simulink model "Main_C0_C3"  (R2023a)
settings: Solver=ode15s  StartTime=0.0  StopTime=1  RelTol=1e-3
model workspace (MAT data in the model file):
  C_IVD = 0.05
  E_IVD1 = 2.1
  E_IVD2 = 2.2
  E_IVD3 = 1.1
  E_IVD4 = 1.7
  E_IVD5 = 3.2
  IVD1 : object (value not decoded)
  IVD2 : object (value not decoded)
  IVD3 : object (value not decoded)
  IVD4 : object (value not decoded)
  IVD5 : object (value not decoded)
  eo_color = [1 0 0]
  io_color = [0 1 0]
  longissimus_color = [1 0 1]
  multifidus_color = [0 1 1]
  muscle_radius = 1
  psoas_color = [0 0 1]
  ra_color = [1 1 0.5]
symbols that are objects in the model workspace (value not decoded): IVD1, IVD2, IVD3, IVD4, IVD5
undefined symbols (not defined in the file or in its folder): AbdFlex, E_TLFflex, IAP_activation_AbdFlex, IAP_Pa, LeftAbdominalMuscleForce, LeftBackMuscleForce, LeftTransverse1MuscleForce, LeftTransverse2MuscleForce, RightAbdominalMuscleForce, RightBackMuscleForce, RightTransverse1MuscleForce, RightTransverse2MuscleForce, TLFflex2, X, Y, Z
libraries: nesl_utility x1235, sm_lib x960, fl_lib x6, simulink_extras x2
(part 33 of 37)

== matlab function Main_C0_C3/Supraspinous Ligaments/SSL Visualization/Ligament3/MATLAB Function2 ==
  data: x1 input; length output; y1 input; z1 input; x2 input; y2 input; z2 input; Rx output; Ry output; Rz output
function [length, Rx, Ry, Rz] = computeCylinderParameters(x1, y1, z1, x2, y2, z2)
    % Compute the vector between the two frames
    vector = [x2 - x1, y2 - y1, z2 - z1];
    
    % Compute the length of the cylinder
    length = norm(vector);
    
    % Normalize the vector for direction
    unit_vector = vector / length;
    
    % Assume fixed axis (Z-axis)
    fixed_axis = [0, 0, 1];
    
    % Compute the axis of rotation (cross product)
    axis_of_rotation = cross(unit_vector, fixed_axis);
    
    % Avoid division by zero in case vectors are parallel
    if norm(axis_of_rotation) == 0
        % Handle case when the vectors are parallel
        if dot(unit_vector, fixed_axis) > 0
            % Vectors are aligned, no rotation needed
            Rx = 0;
            Ry = 0;
            Rz = 0;
        else
            % Vectors are in opposite directions, 180 degree rotation
            Rx = pi;
            Ry = 0;
            Rz = 0;
        end
        return;
    end
    
    % Normalize the axis of rotation
    axis_of_rotation = axis_of_rotation / norm(axis_of_rotation);
    
    % Compute the angle between vectors (dot product)
    cos_theta = dot(unit_vector, fixed_axis);
    
    % Clamp cos_theta to the range [-1, 1] to avoid domain errors in acos
    cos_theta = max(min(cos_theta, 1), -1);
    angle = acos(cos_theta);  % The angle between the vectors
    
    % Rodrigues' rotation formula to compute the rotation matrix
    K = [0, -axis_of_rotation(3), axis_of_rotation(2); 
         axis_of_rotation(3), 0, -axis_of_rotation(1); 
         -axis_of_rotation(2), axis_of_rotation(1), 0]; 
    R = eye(3) + sin(angle)*K + (1 - cos(angle))*(K^2);
    
    % Now, decompose the rotation matrix to extract the Euler angles
    Rx = -atan2(R(3,2), R(3,3)); % Rotation about X-axis
    %Ry = atan2(-R(3,1), sqrt(R(3,2)^2 + R(3,3)^2)); % Rotation about Y-axis
    denominator = max(sqrt(R(3,2)^2 + R(3,3)^2), eps); % Avoid division by zero
    Ry = -atan2(-R(3,1), denominator);

    
    
    Rz = 0; % No additional rotation needed around the Z-axis
end

== matlab function Main_C0_C3/Muscle Forces/Muscle Visualization/Psoas Visualization/Muscle8/MATLAB Function2 ==
  data: x1 input; length output; y1 input; z1 input; x2 input; y2 input; z2 input; Rx output; Ry output; Rz output
function [length, Rx, Ry, Rz] = computeCylinderParameters(x1, y1, z1, x2, y2, z2)
    % Compute the vector between the two frames
    vector = [x2 - x1, y2 - y1, z2 - z1];
    
    % Compute the length of the cylinder
    length = norm(vector);
    
    % Normalize the vector for direction
    unit_vector = vector / length;
    
    % Assume fixed axis (Z-axis)
    fixed_axis = [0, 0, 1];
    
    % Compute the axis of rotation (cross product)
    axis_of_rotation = cross(unit_vector, fixed_axis);
    
    % Avoid division by zero in case vectors are parallel
    if norm(axis_of_rotation) == 0
        % Handle case when the vectors are parallel
        if dot(unit_vector, fixed_axis) > 0
            % Vectors are aligned, no rotation needed
            Rx = 0;
            Ry = 0;
            Rz = 0;
        else
            % Vectors are in opposite directions, 180 degree rotation
            Rx = pi;
            Ry = 0;
            Rz = 0;
        end
        return;
    end
    
    % Normalize the axis of rotation
    axis_of_rotation = axis_of_rotation / norm(axis_of_rotation);
    
    % Compute the angle between vectors (dot product)
    cos_theta = dot(unit_vector, fixed_axis);
    
    % Clamp cos_theta to the range [-1, 1] to avoid domain errors in acos
    cos_theta = max(min(cos_theta, 1), -1);
    angle = acos(cos_theta);  % The angle between the vectors
    
    % Rodrigues' rotation formula to compute the rotation matrix
    K = [0, -axis_of_rotation(3), axis_of_rotation(2); 
         axis_of_rotation(3), 0, -axis_of_rotation(1); 
         -axis_of_rotation(2), axis_of_rotation(1), 0]; 
    R = eye(3) + sin(angle)*K + (1 - cos(angle))*(K^2);
    
    % Now, decompose the rotation matrix to extract the Euler angles
    Rx = -atan2(R(3,2), R(3,3)); % Rotation about X-axis
    %Ry = atan2(-R(3,1), sqrt(R(3,2)^2 + R(3,3)^2)); % Rotation about Y-axis
    denominator = max(sqrt(R(3,2)^2 + R(3,3)^2), eps); % Avoid division by zero
    Ry = -atan2(-R(3,1), denominator);

    
    
    Rz = 0; % No additional rotation needed around the Z-axis
end

== matlab function Main_C0_C3/Supraspinous Ligaments/SSL Visualization/Ligament4/MATLAB Function2 ==
  data: x1 input; length output; y1 input; z1 input; x2 input; y2 input; z2 input; Rx output; Ry output; Rz output
function [length, Rx, Ry, Rz] = computeCylinderParameters(x1, y1, z1, x2, y2, z2)
    % Compute the vector between the two frames
    vector = [x2 - x1, y2 - y1, z2 - z1];
    
    % Compute the length of the cylinder
    length = norm(vector);
    
    % Normalize the vector for direction
    unit_vector = vector / length;
    
    % Assume fixed axis (Z-axis)
    fixed_axis = [0, 0, 1];
    
    % Compute the axis of rotation (cross product)
    axis_of_rotation = cross(unit_vector, fixed_axis);
    
    % Avoid division by zero in case vectors are parallel
    if norm(axis_of_rotation) == 0
        % Handle case when the vectors are parallel
        if dot(unit_vector, fixed_axis) > 0
            % Vectors are aligned, no rotation needed
            Rx = 0;
            Ry = 0;
            Rz = 0;
        else
            % Vectors are in opposite directions, 180 degree rotation
            Rx = pi;
            Ry = 0;
            Rz = 0;
        end
        return;
    end
    
    % Normalize the axis of rotation
    axis_of_rotation = axis_of_rotation / norm(axis_of_rotation);
    
    % Compute the angle between vectors (dot product)
    cos_theta = dot(unit_vector, fixed_axis);
    
    % Clamp cos_theta to the range [-1, 1] to avoid domain errors in acos
    cos_theta = max(min(cos_theta, 1), -1);
    angle = acos(cos_theta);  % The angle between the vectors
    
    % Rodrigues' rotation formula to compute the rotation matrix
    K = [0, -axis_of_rotation(3), axis_of_rotation(2); 
         axis_of_rotation(3), 0, -axis_of_rotation(1); 
         -axis_of_rotation(2), axis_of_rotation(1), 0]; 
    R = eye(3) + sin(angle)*K + (1 - cos(angle))*(K^2);
    
    % Now, decompose the rotation matrix to extract the Euler angles
    Rx = -atan2(R(3,2), R(3,3)); % Rotation about X-axis
    %Ry = atan2(-R(3,1), sqrt(R(3,2)^2 + R(3,3)^2)); % Rotation about Y-axis
    denominator = max(sqrt(R(3,2)^2 + R(3,3)^2), eps); % Avoid division by zero
    Ry = -atan2(-R(3,1), denominator);

    
    
    Rz = 0; % No additional rotation needed around the Z-axis
end

== matlab function Main_C0_C3/Left and Right Intertransverse Ligaments/ITL Visualization - debug/Ligament3/MATLAB Function2 ==
  data: x1 input; length output; y1 input; z1 input; x2 input; y2 input; z2 input; Rx output; Ry output; Rz output
function [length, Rx, Ry, Rz] = computeCylinderParameters(x1, y1, z1, x2, y2, z2)
    % Compute the vector between the two frames
    vector = [x2 - x1, y2 - y1, z2 - z1];
    
    % Compute the length of the cylinder
    length = norm(vector);
    
    % Normalize the vector for direction
    unit_vector = vector / length;
    
    % Assume fixed axis (Z-axis)
    fixed_axis = [0, 0, 1];
    
    % Compute the axis of rotation (cross product)
    axis_of_rotation = cross(unit_vector, fixed_axis);
    
    % Avoid division by zero in case vectors are parallel
    if norm(axis_of_rotation) == 0
        % Handle case when the vectors are parallel
        if dot(unit_vector, fixed_axis) > 0
            % Vectors are aligned, no rotation needed
            Rx = 0;
            Ry = 0;
            Rz = 0;
        else
            % Vectors are in opposite directions, 180 degree rotation
            Rx = pi;
            Ry = 0;
            Rz = 0;
        end
        return;
    end
    
    % Normalize the axis of rotation
    axis_of_rotation = axis_of_rotation / norm(axis_of_rotation);
    
    % Compute the angle between vectors (dot product)
    cos_theta = dot(unit_vector, fixed_axis);
    
    % Clamp cos_theta to the range [-1, 1] to avoid domain errors in acos
    cos_theta = max(min(cos_theta, 1), -1);
    angle = acos(cos_theta);  % The angle between the vectors
    
    % Rodrigues' rotation formula to compute the rotation matrix
    K = [0, -axis_of_rotation(3), axis_of_rotation(2); 
         axis_of_rotation(3), 0, -axis_of_rotation(1); 
         -axis_of_rotation(2), axis_of_rotation(1), 0]; 
    R = eye(3) + sin(angle)*K + (1 - cos(angle))*(K^2);
    
    % Now, decompose the rotation matrix to extract the Euler angles
    Rx = -atan2(R(3,2), R(3,3)); % Rotation about X-axis
    %Ry = atan2(-R(3,1), sqrt(R(3,2)^2 + R(3,3)^2)); % Rotation about Y-axis
    denominator = max(sqrt(R(3,2)^2 + R(3,3)^2), eps); % Avoid division by zero
    Ry = -atan2(-R(3,1), denominator);

    
    
    Rz = 0; % No additional rotation needed around the Z-axis
end

== matlab function Main_C0_C3/Left and Right Intertransverse Ligaments/ITL Visualization - debug/Ligament1/MATLAB Function2 ==
  data: x1 input; length output; y1 input; z1 input; x2 input; y2 input; z2 input; Rx output; Ry output; Rz output
function [length, Rx, Ry, Rz] = computeCylinderParameters(x1, y1, z1, x2, y2, z2)
    % Compute the vector between the two frames
    vector = [x2 - x1, y2 - y1, z2 - z1];
    
    % Compute the length of the cylinder
    length = norm(vector);
    
    % Normalize the vector for direction
    unit_vector = vector / length;
    
    % Assume fixed axis (Z-axis)
    fixed_axis = [0, 0, 1];
    
    % Compute the axis of rotation (cross product)
    axis_of_rotation = cross(unit_vector, fixed_axis);
    
    % Avoid division by zero in case vectors are parallel
    if norm(axis_of_rotation) == 0
        % Handle case when the vectors are parallel
        if dot(unit_vector, fixed_axis) > 0
            % Vectors are aligned, no rotation needed
            Rx = 0;
            Ry = 0;
            Rz = 0;
        else
            % Vectors are in opposite directions, 180 degree rotation
            Rx = pi;
            Ry = 0;
            Rz = 0;
        end
        return;
    end
    
    % Normalize the axis of rotation
    axis_of_rotation = axis_of_rotation / norm(axis_of_rotation);
    
    % Compute the angle between vectors (dot product)
    cos_theta = dot(unit_vector, fixed_axis);
    
    % Clamp cos_theta to the range [-1, 1] to avoid domain errors in acos
    cos_theta = max(min(cos_theta, 1), -1);
    angle = acos(cos_theta);  % The angle between the vectors
    
    % Rodrigues' rotation formula to compute the rotation matrix
    K = [0, -axis_of_rotation(3), axis_of_rotation(2); 
         axis_of_rotation(3), 0, -axis_of_rotation(1); 
         -axis_of_rotation(2), axis_of_rotation(1), 0]; 
    R = eye(3) + sin(angle)*K + (1 - cos(angle))*(K^2);
    
    % Now, decompose the rotation matrix to extract the Euler angles
    Rx = -atan2(R(3,2), R(3,3)); % Rotation about X-axis
    %Ry = atan2(-R(3,1), sqrt(R(3,2)^2 + R(3,3)^2)); % Rotation about Y-axis
    denominator = max(sqrt(R(3,2)^2 + R(3,3)^2), eps); % Avoid division by zero
    Ry = -atan2(-R(3,1), denominator);

    
    
    Rz = 0; % No additional rotation needed around the Z-axis
end

== matlab function Main_C0_C3/Left and Right Intertransverse Ligaments/ITL Visualization - debug/Ligament2/MATLAB Function2 ==
  data: x1 input; length output; y1 input; z1 input; x2 input; y2 input; z2 input; Rx output; Ry output; Rz output
function [length, Rx, Ry, Rz] = computeCylinderParameters(x1, y1, z1, x2, y2, z2)
    % Compute the vector between the two frames
    vector = [x2 - x1, y2 - y1, z2 - z1];
    
    % Compute the length of the cylinder
    length = norm(vector);
    
    % Normalize the vector for direction
    unit_vector = vector / length;
    
    % Assume fixed axis (Z-axis)
    fixed_axis = [0, 0, 1];
    
    % Compute the axis of rotation (cross product)
    axis_of_rotation = cross(unit_vector, fixed_axis);
    
    % Avoid division by zero in case vectors are parallel
    if norm(axis_of_rotation) == 0
        % Handle case when the vectors are parallel
        if dot(unit_vector, fixed_axis) > 0
            % Vectors are aligned, no rotation needed
            Rx = 0;
            Ry = 0;
            Rz = 0;
        else
            % Vectors are in opposite directions, 180 degree rotation
            Rx = pi;
            Ry = 0;
            Rz = 0;
        end
        return;
    end
    
    % Normalize the axis of rotation
    axis_of_rotation = axis_of_rotation / norm(axis_of_rotation);
    
    % Compute the angle between vectors (dot product)
    cos_theta = dot(unit_vector, fixed_axis);
    
    % Clamp cos_theta to the range [-1, 1] to avoid domain errors in acos
    cos_theta = max(min(cos_theta, 1), -1);
    angle = acos(cos_theta);  % The angle between the vectors
    
    % Rodrigues' rotation formula to compute the rotation matrix
    K = [0, -axis_of_rotation(3), axis_of_rotation(2); 
         axis_of_rotation(3), 0, -axis_of_rotation(1); 
         -axis_of_rotation(2), axis_of_rotation(1), 0]; 
    R = eye(3) + sin(angle)*K + (1 - cos(angle))*(K^2);
    
    % Now, decompose the rotation matrix to extract the Euler angles
    Rx = -atan2(R(3,2), R(3,3)); % Rotation about X-axis
    %Ry = atan2(-R(3,1), sqrt(R(3,2)^2 + R(3,3)^2)); % Rotation about Y-axis
    denominator = max(sqrt(R(3,2)^2 + R(3,3)^2), eps); % Avoid division by zero
    Ry = -atan2(-R(3,1), denominator);

    
    
    Rz = 0; % No additional rotation needed around the Z-axis
end

== matlab function Main_C0_C3/Left and Right Intertransverse Ligaments/ITL Visualization - debug/Ligament4/MATLAB Function2 ==
  data: x1 input; length output; y1 input; z1 input; x2 input; y2 input; z2 input; Rx output; Ry output; Rz output
function [length, Rx, Ry, Rz] = computeCylinderParameters(x1, y1, z1, x2, y2, z2)
    % Compute the vector between the two frames
    vector = [x2 - x1, y2 - y1, z2 - z1];
    
    % Compute the length of the cylinder
    length = norm(vector);
    
    % Normalize the vector for direction
    unit_vector = vector / length;
    
    % Assume fixed axis (Z-axis)
    fixed_axis = [0, 0, 1];
    
    % Compute the axis of rotation (cross product)
    axis_of_rotation = cross(unit_vector, fixed_axis);
    
    % Avoid division by zero in case vectors are parallel
    if norm(axis_of_rotation) == 0
        % Handle case when the vectors are parallel
        if dot(unit_vector, fixed_axis) > 0
            % Vectors are aligned, no rotation needed
            Rx = 0;
            Ry = 0;
            Rz = 0;
        else
            % Vectors are in opposite directions, 180 degree rotation
            Rx = pi;
            Ry = 0;
            Rz = 0;
        end
        return;
    end
    
    % Normalize the axis of rotation
    axis_of_rotation = axis_of_rotation / norm(axis_of_rotation);
    
    % Compute the angle between vectors (dot product)
    cos_theta = dot(unit_vector, fixed_axis);
    
    % Clamp cos_theta to the range [-1, 1] to avoid domain errors in acos
    cos_theta = max(min(cos_theta, 1), -1);
    angle = acos(cos_theta);  % The angle between the vectors
    
    % Rodrigues' rotation formula to compute the rotation matrix
    K = [0, -axis_of_rotation(3), axis_of_rotation(2); 
         axis_of_rotation(3), 0, -axis_of_rotation(1); 
         -axis_of_rotation(2), axis_of_rotation(1), 0]; 
    R = eye(3) + sin(angle)*K + (1 - cos(angle))*(K^2);
    
    % Now, decompose the rotation matrix to extract the Euler angles
    Rx = -atan2(R(3,2), R(3,3)); % Rotation about X-axis
    %Ry = atan2(-R(3,1), sqrt(R(3,2)^2 + R(3,3)^2)); % Rotation about Y-axis
    denominator = max(sqrt(R(3,2)^2 + R(3,3)^2), eps); % Avoid division by zero
    Ry = -atan2(-R(3,1), denominator);

    
    
    Rz = 0; % No additional rotation needed around the Z-axis
end

== matlab function Main_C0_C3/Left and Right Intertransverse Ligaments/ITL Visualization - debug/Ligament5/MATLAB Function2 ==
  data: x1 input; length output; y1 input; z1 input; x2 input; y2 input; z2 input; Rx output; Ry output; Rz output
function [length, Rx, Ry, Rz] = computeCylinderParameters(x1, y1, z1, x2, y2, z2)
    % Compute the vector between the two frames
    vector = [x2 - x1, y2 - y1, z2 - z1];
    
    % Compute the length of the cylinder
    length = norm(vector);
    
    % Normalize the vector for direction
    unit_vector = vector / length;
    
    % Assume fixed axis (Z-axis)
    fixed_axis = [0, 0, 1];
    
    % Compute the axis of rotation (cross product)
    axis_of_rotation = cross(unit_vector, fixed_axis);
    
    % Avoid division by zero in case vectors are parallel
    if norm(axis_of_rotation) == 0
        % Handle case when the vectors are parallel
        if dot(unit_vector, fixed_axis) > 0
            % Vectors are aligned, no rotation needed
            Rx = 0;
            Ry = 0;
            Rz = 0;
        else
            % Vectors are in opposite directions, 180 degree rotation
            Rx = pi;
            Ry = 0;
            Rz = 0;
        end
        return;
    end
    
    % Normalize the axis of rotation
    axis_of_rotation = axis_of_rotation / norm(axis_of_rotation);
    
    % Compute the angle between vectors (dot product)
    cos_theta = dot(unit_vector, fixed_axis);
    
    % Clamp cos_theta to the range [-1, 1] to avoid domain errors in acos
    cos_theta = max(min(cos_theta, 1), -1);
    angle = acos(cos_theta);  % The angle between the vectors
    
    % Rodrigues' rotation formula to compute the rotation matrix
    K = [0, -axis_of_rotation(3), axis_of_rotation(2); 
         axis_of_rotation(3), 0, -axis_of_rotation(1); 
         -axis_of_rotation(2), axis_of_rotation(1), 0]; 
    R = eye(3) + sin(angle)*K + (1 - cos(angle))*(K^2);
    
    % Now, decompose the rotation matrix to extract the Euler angles
    Rx = -atan2(R(3,2), R(3,3)); % Rotation about X-axis
    %Ry = atan2(-R(3,1), sqrt(R(3,2)^2 + R(3,3)^2)); % Rotation about Y-axis
    denominator = max(sqrt(R(3,2)^2 + R(3,3)^2), eps); % Avoid division by zero
    Ry = -atan2(-R(3,1), denominator);

    
    
    Rz = 0; % No additional rotation needed around the Z-axis
end

== matlab function Main_C0_C3/Left and Right Intertransverse Ligaments/ITL Visualization - debug/Ligament6/MATLAB Function2 ==
  data: x1 input; length output; y1 input; z1 input; x2 input; y2 input; z2 input; Rx output; Ry output; Rz output
function [length, Rx, Ry, Rz] = computeCylinderParameters(x1, y1, z1, x2, y2, z2)
    % Compute the vector between the two frames
    vector = [x2 - x1, y2 - y1, z2 - z1];
    
    % Compute the length of the cylinder
    length = norm(vector);
    
    % Normalize the vector for direction
    unit_vector = vector / length;
    
    % Assume fixed axis (Z-axis)
    fixed_axis = [0, 0, 1];
    
    % Compute the axis of rotation (cross product)
    axis_of_rotation = cross(unit_vector, fixed_axis);
    
    % Avoid division by zero in case vectors are parallel
    if norm(axis_of_rotation) == 0
        % Handle case when the vectors are parallel
        if dot(unit_vector, fixed_axis) > 0
            % Vectors are aligned, no rotation needed
            Rx = 0;
            Ry = 0;
            Rz = 0;
        else
            % Vectors are in opposite directions, 180 degree rotation
            Rx = pi;
            Ry = 0;
            Rz = 0;
        end
        return;
    end
    
    % Normalize the axis of rotation
    axis_of_rotation = axis_of_rotation / norm(axis_of_rotation);
    
    % Compute the angle between vectors (dot product)
    cos_theta = dot(unit_vector, fixed_axis);
    
    % Clamp cos_theta to the range [-1, 1] to avoid domain errors in acos
    cos_theta = max(min(cos_theta, 1), -1);
    angle = acos(cos_theta);  % The angle between the vectors
    
    % Rodrigues' rotation formula to compute the rotation matrix
    K = [0, -axis_of_rotation(3), axis_of_rotation(2); 
         axis_of_rotation(3), 0, -axis_of_rotation(1); 
         -axis_of_rotation(2), axis_of_rotation(1), 0]; 
    R = eye(3) + sin(angle)*K + (1 - cos(angle))*(K^2);
    
    % Now, decompose the rotation matrix to extract the Euler angles
    Rx = -atan2(R(3,2), R(3,3)); % Rotation about X-axis
    %Ry = atan2(-R(3,1), sqrt(R(3,2)^2 + R(3,3)^2)); % Rotation about Y-axis
    denominator = max(sqrt(R(3,2)^2 + R(3,3)^2), eps); % Avoid division by zero
    Ry = -atan2(-R(3,1), denominator);

    
    
    Rz = 0; % No additional rotation needed around the Z-axis
end

== matlab function Main_C0_C3/Left and Right Intertransverse Ligaments/ITL Visualization - debug/Ligament7/MATLAB Function2 ==
  data: x1 input; length output; y1 input; z1 input; x2 input; y2 input; z2 input; Rx output; Ry output; Rz output
function [length, Rx, Ry, Rz] = computeCylinderParameters(x1, y1, z1, x2, y2, z2)
    % Compute the vector between the two frames
    vector = [x2 - x1, y2 - y1, z2 - z1];
    
    % Compute the length of the cylinder
    length = norm(vector);
    
    % Normalize the vector for direction
    unit_vector = vector / length;
    
    % Assume fixed axis (Z-axis)
    fixed_axis = [0, 0, 1];
    
    % Compute the axis of rotation (cross product)
    axis_of_rotation = cross(unit_vector, fixed_axis);
    
    % Avoid division by zero in case vectors are parallel
    if norm(axis_of_rotation) == 0
        % Handle case when the vectors are parallel
        if dot(unit_vector, fixed_axis) > 0
            % Vectors are aligned, no rotation needed
            Rx = 0;
            Ry = 0;
            Rz = 0;
        else
            % Vectors are in opposite directions, 180 degree rotation
            Rx = pi;
            Ry = 0;
            Rz = 0;
        end
        return;
    end
    
    % Normalize the axis of rotation
    axis_of_rotation = axis_of_rotation / norm(axis_of_rotation);
    
    % Compute the angle between vectors (dot product)
    cos_theta = dot(unit_vector, fixed_axis);
    
    % Clamp cos_theta to the range [-1, 1] to avoid domain errors in acos
    cos_theta = max(min(cos_theta, 1), -1);
    angle = acos(cos_theta);  % The angle between the vectors
    
    % Rodrigues' rotation formula to compute the rotation matrix
    K = [0, -axis_of_rotation(3), axis_of_rotation(2); 
         axis_of_rotation(3), 0, -axis_of_rotation(1); 
         -axis_of_rotation(2), axis_of_rotation(1), 0]; 
    R = eye(3) + sin(angle)*K + (1 - cos(angle))*(K^2);
    
    % Now, decompose the rotation matrix to extract the Euler angles
    Rx = -atan2(R(3,2), R(3,3)); % Rotation about X-axis
    %Ry = atan2(-R(3,1), sqrt(R(3,2)^2 + R(3,3)^2)); % Rotation about Y-axis
    denominator = max(sqrt(R(3,2)^2 + R(3,3)^2), eps); % Avoid division by zero
    Ry = -atan2(-R(3,1), denominator);

    
    
    Rz = 0; % No additional rotation needed around the Z-axis
end

== matlab function Main_C0_C3/Left and Right Intertransverse Ligaments/ITL Visualization - debug/Ligament8/MATLAB Function2 ==
  data: x1 input; length output; y1 input; z1 input; x2 input; y2 input; z2 input; Rx output; Ry output; Rz output
function [length, Rx, Ry, Rz] = computeCylinderParameters(x1, y1, z1, x2, y2, z2)
    % Compute the vector between the two frames
    vector = [x2 - x1, y2 - y1, z2 - z1];
    
    % Compute the length of the cylinder
    length = norm(vector);
    
    % Normalize the vector for direction
    unit_vector = vector / length;
    
    % Assume fixed axis (Z-axis)
    fixed_axis = [0, 0, 1];
    
    % Compute the axis of rotation (cross product)
    axis_of_rotation = cross(unit_vector, fixed_axis);
    
    % Avoid division by zero in case vectors are parallel
    if norm(axis_of_rotation) == 0
        % Handle case when the vectors are parallel
        if dot(unit_vector, fixed_axis) > 0
            % Vectors are aligned, no rotation needed
            Rx = 0;
            Ry = 0;
            Rz = 0;
        else
            % Vectors are in opposite directions, 180 degree rotation
            Rx = pi;
            Ry = 0;
            Rz = 0;
        end
        return;
    end
    
    % Normalize the axis of rotation
    axis_of_rotation = axis_of_rotation / norm(axis_of_rotation);
    
    % Compute the angle between vectors (dot product)
    cos_theta = dot(unit_vector, fixed_axis);
    
    % Clamp cos_theta to the range [-1, 1] to avoid domain errors in acos
    cos_theta = max(min(cos_theta, 1), -1);
    angle = acos(cos_theta);  % The angle between the vectors
    
    % Rodrigues' rotation formula to compute the rotation matrix
    K = [0, -axis_of_rotation(3), axis_of_rotation(2); 
         axis_of_rotation(3), 0, -axis_of_rotation(1); 
         -axis_of_rotation(2), axis_of_rotation(1), 0]; 
    R = eye(3) + sin(angle)*K + (1 - cos(angle))*(K^2);
    
    % Now, decompose the rotation matrix to extract the Euler angles
    Rx = -atan2(R(3,2), R(3,3)); % Rotation about X-axis
    %Ry = atan2(-R(3,1), sqrt(R(3,2)^2 + R(3,3)^2)); % Rotation about Y-axis
    denominator = max(sqrt(R(3,2)^2 + R(3,3)^2), eps); % Avoid division by zero
    Ry = -atan2(-R(3,1), denominator);

    
    
    Rz = 0; % No additional rotation needed around the Z-axis
end

== matlab function Main_C0_C3/Left and Right Intertransverse Ligaments/ITL Visualization - debug/Ligament9/MATLAB Function2 ==
  data: x1 input; length output; y1 input; z1 input; x2 input; y2 input; z2 input; Rx output; Ry output; Rz output
function [length, Rx, Ry, Rz] = computeCylinderParameters(x1, y1, z1, x2, y2, z2)
    % Compute the vector between the two frames
    vector = [x2 - x1, y2 - y1, z2 - z1];
    
    % Compute the length of the cylinder
    length = norm(vector);
    
    % Normalize the vector for direction
    unit_vector = vector / length;
    
    % Assume fixed axis (Z-axis)
    fixed_axis = [0, 0, 1];
    
    % Compute the axis of rotation (cross product)
    axis_of_rotation = cross(unit_vector, fixed_axis);
    
    % Avoid division by zero in case vectors are parallel
    if norm(axis_of_rotation) == 0
        % Handle case when the vectors are parallel
        if dot(unit_vector, fixed_axis) > 0
            % Vectors are aligned, no rotation needed
            Rx = 0;
            Ry = 0;
            Rz = 0;
        else
            % Vectors are in opposite directions, 180 degree rotation
            Rx = pi;
            Ry = 0;
            Rz = 0;
        end
        return;
    end
    
    % Normalize the axis of rotation
    axis_of_rotation = axis_of_rotation / norm(axis_of_rotation);
    
    % Compute the angle between vectors (dot product)
    cos_theta = dot(unit_vector, fixed_axis);
    
    % Clamp cos_theta to the range [-1, 1] to avoid domain errors in acos
    cos_theta = max(min(cos_theta, 1), -1);
    angle = acos(cos_theta);  % The angle between the vectors
    
    % Rodrigues' rotation formula to compute the rotation matrix
    K = [0, -axis_of_rotation(3), axis_of_rotation(2); 
         axis_of_rotation(3), 0, -axis_of_rotation(1); 
         -axis_of_rotation(2), axis_of_rotation(1), 0]; 
    R = eye(3) + sin(angle)*K + (1 - cos(angle))*(K^2);
    
    % Now, decompose the rotation matrix to extract the Euler angles
    Rx = -atan2(R(3,2), R(3,3)); % Rotation about X-axis
    %Ry = atan2(-R(3,1), sqrt(R(3,2)^2 + R(3,3)^2)); % Rotation about Y-axis
    denominator = max(sqrt(R(3,2)^2 + R(3,3)^2), eps); % Avoid division by zero
    Ry = -atan2(-R(3,1), denominator);

    
    
    Rz = 0; % No additional rotation needed around the Z-axis
end

== matlab function Main_C0_C3/Muscle Forces/Muscle Visualization/Multifidus Visualization/Muscle9/MATLAB Function2 ==
  data: x1 input; length output; y1 input; z1 input; x2 input; y2 input; z2 input; Rx output; Ry output; Rz output
function [length, Rx, Ry, Rz] = computeCylinderParameters(x1, y1, z1, x2, y2, z2)
    % Compute the vector between the two frames
    vector = [x2 - x1, y2 - y1, z2 - z1];
    
    % Compute the length of the cylinder
    length = norm(vector);
    
    % Normalize the vector for direction
    unit_vector = vector / length;
    
    % Assume fixed axis (Z-axis)
    fixed_axis = [0, 0, 1];
    
    % Compute the axis of rotation (cross product)
    axis_of_rotation = cross(unit_vector, fixed_axis);
    
    % Avoid division by zero in case vectors are parallel
    if norm(axis_of_rotation) == 0
        % Handle case when the vectors are parallel
        if dot(unit_vector, fixed_axis) > 0
            % Vectors are aligned, no rotation needed
            Rx = 0;
            Ry = 0;
            Rz = 0;
        else
            % Vectors are in opposite directions, 180 degree rotation
            Rx = pi;
            Ry = 0;
            Rz = 0;
        end
        return;
    end
    
    % Normalize the axis of rotation
    axis_of_rotation = axis_of_rotation / norm(axis_of_rotation);
    
    % Compute the angle between vectors (dot product)
    cos_theta = dot(unit_vector, fixed_axis);
    
    % Clamp cos_theta to the range [-1, 1] to avoid domain errors in acos
    cos_theta = max(min(cos_theta, 1), -1);
    angle = acos(cos_theta);  % The angle between the vectors
    
    % Rodrigues' rotation formula to compute the rotation matrix
    K = [0, -axis_of_rotation(3), axis_of_rotation(2); 
         axis_of_rotation(3), 0, -axis_of_rotation(1); 
         -axis_of_rotation(2), axis_of_rotation(1), 0]; 
    R = eye(3) + sin(angle)*K + (1 - cos(angle))*(K^2);
    
    % Now, decompose the rotation matrix to extract the Euler angles
    Rx = -atan2(R(3,2), R(3,3)); % Rotation about X-axis
    %Ry = atan2(-R(3,1), sqrt(R(3,2)^2 + R(3,3)^2)); % Rotation about Y-axis
    denominator = max(sqrt(R(3,2)^2 + R(3,3)^2), eps); % Avoid division by zero
    Ry = -atan2(-R(3,1), denominator);

    
    
    Rz = 0; % No additional rotation needed around the Z-axis
end

== matlab function Main_C0_C3/Left and Right Intertransverse Ligaments/ITL Visualization - debug/Ligament10/MATLAB Function2 ==
  data: x1 input; length output; y1 input; z1 input; x2 input; y2 input; z2 input; Rx output; Ry output; Rz output
function [length, Rx, Ry, Rz] = computeCylinderParameters(x1, y1, z1, x2, y2, z2)
    % Compute the vector between the two frames
    vector = [x2 - x1, y2 - y1, z2 - z1];
    
    % Compute the length of the cylinder
    length = norm(vector);
    
    % Normalize the vector for direction
    unit_vector = vector / length;
    
    % Assume fixed axis (Z-axis)
    fixed_axis = [0, 0, 1];
    
    % Compute the axis of rotation (cross product)
    axis_of_rotation = cross(unit_vector, fixed_axis);
    
    % Avoid division by zero in case vectors are parallel
    if norm(axis_of_rotation) == 0
        % Handle case when the vectors are parallel
        if dot(unit_vector, fixed_axis) > 0
            % Vectors are aligned, no rotation needed
            Rx = 0;
            Ry = 0;
            Rz = 0;
        else
            % Vectors are in opposite directions, 180 degree rotation
            Rx = pi;
            Ry = 0;
            Rz = 0;
        end
        return;
    end
    
    % Normalize the axis of rotation
    axis_of_rotation = axis_of_rotation / norm(axis_of_rotation);
    
    % Compute the angle between vectors (dot product)
    cos_theta = dot(unit_vector, fixed_axis);
    
    % Clamp cos_theta to the range [-1, 1] to avoid domain errors in acos
    cos_theta = max(min(cos_theta, 1), -1);
    angle = acos(cos_theta);  % The angle between the vectors
    
    % Rodrigues' rotation formula to compute the rotation matrix
    K = [0, -axis_of_rotation(3), axis_of_rotation(2); 
         axis_of_rotation(3), 0, -axis_of_rotation(1); 
         -axis_of_rotation(2), axis_of_rotation(1), 0]; 
    R = eye(3) + sin(angle)*K + (1 - cos(angle))*(K^2);
    
    % Now, decompose the rotation matrix to extract the Euler angles
    Rx = -atan2(R(3,2), R(3,3)); % Rotation about X-axis
    %Ry = atan2(-R(3,1), sqrt(R(3,2)^2 + R(3,3)^2)); % Rotation about Y-axis
    denominator = max(sqrt(R(3,2)^2 + R(3,3)^2), eps); % Avoid division by zero
    Ry = -atan2(-R(3,1), denominator);

    
    
    Rz = 0; % No additional rotation needed around the Z-axis
end

== matlab function Main_C0_C3/TLF Flex/Latissimus Dorsi/WrappedMuscle2/MATLAB Function1 ==
  data: x1 input; length output; y1 input; z1 input; x2 input; y2 input; z2 input; Rx output; Ry output; Rz output
function [length, Rx, Ry, Rz] = computeCylinderParameters(x1, y1, z1, x2, y2, z2)
    % Compute the vector between the two frames
    vector = [x2 - x1, y2 - y1, z2 - z1];
    
    % Compute the length of the cylinder
    length = norm(vector);
    
    % Normalize the vector for direction
    unit_vector = vector / length;
    
    % Assume fixed axis (Z-axis)
    fixed_axis = [0, 0, 1];
    
    % Compute the axis of rotation (cross product)
    axis_of_rotation = cross(unit_vector, fixed_axis);
    
    % Avoid division by zero in case vectors are parallel
    if norm(axis_of_rotation) == 0
        % Handle case when the vectors are parallel
        if dot(unit_vector, fixed_axis) > 0
            % Vectors are aligned, no rotation needed
            Rx = 0;
            Ry = 0;
            Rz = 0;
        else
            % Vectors are in opposite directions, 180 degree rotation
            Rx = pi;
            Ry = 0;
            Rz = 0;
        end
        return;
    end
    
    % Normalize the axis of rotation
    axis_of_rotation = axis_of_rotation / norm(axis_of_rotation);
    
    % Compute the angle between vectors (dot product)
    cos_theta = dot(unit_vector, fixed_axis);
    
    % Clamp cos_theta to the range [-1, 1] to avoid domain errors in acos
    cos_theta = max(min(cos_theta, 1), -1);
    angle = acos(cos_theta);  % The angle between the vectors
    
    % Rodrigues' rotation formula to compute the rotation matrix
    K = [0, -axis_of_rotation(3), axis_of_rotation(2); 
         axis_of_rotation(3), 0, -axis_of_rotation(1); 
         -axis_of_rotation(2), axis_of_rotation(1), 0]; 
    R = eye(3) + sin(angle)*K + (1 - cos(angle))*(K^2);
    
    % Now, decompose the rotation matrix to extract the Euler angles
    Rx = -atan2(R(3,2), R(3,3)); % Rotation about X-axis
    %Ry = atan2(-R(3,1), sqrt(R(3,2)^2 + R(3,3)^2)); % Rotation about Y-axis
    denominator = max(sqrt(R(3,2)^2 + R(3,3)^2), eps); % Avoid division by zero
    Ry = -atan2(-R(3,1), denominator);

    
    
    Rz = 0; % No additional rotation needed around the Z-axis
end

== matlab function Main_C0_C3/TLF Flex/Latissimus Dorsi/WrappedMuscle1/MATLAB Function3 ==
  data: x1 input; length output; y1 input; z1 input; x2 input; y2 input; z2 input; Rx output; Ry output; Rz output
function [length, Rx, Ry, Rz] = computeCylinderParameters(x1, y1, z1, x2, y2, z2)
    % Compute the vector between the two frames
    vector = [x2 - x1, y2 - y1, z2 - z1];
    
    % Compute the length of the cylinder
    length = norm(vector);
    
    % Normalize the vector for direction
    unit_vector = vector / length;
    
    % Assume fixed axis (Z-axis)
    fixed_axis = [0, 0, 1];
    
    % Compute the axis of rotation (cross product)
    axis_of_rotation = cross(unit_vector, fixed_axis);
    
    % Avoid division by zero in case vectors are parallel
    if norm(axis_of_rotation) == 0
        % Handle case when the vectors are parallel
        if dot(unit_vector, fixed_axis) > 0
            % Vectors are aligned, no rotation needed
            Rx = 0;
            Ry = 0;
            Rz = 0;
        else
            % Vectors are in opposite directions, 180 degree rotation
            Rx = pi;
            Ry = 0;
            Rz = 0;
        end
        return;
    end
    
    % Normalize the axis of rotation
    axis_of_rotation = axis_of_rotation / norm(axis_of_rotation);
    
    % Compute the angle between vectors (dot product)
    cos_theta = dot(unit_vector, fixed_axis);
    
    % Clamp cos_theta to the range [-1, 1] to avoid domain errors in acos
    cos_theta = max(min(cos_theta, 1), -1);
    angle = acos(cos_theta);  % The angle between the vectors
    
    % Rodrigues' rotation formula to compute the rotation matrix
    K = [0, -axis_of_rotation(3), axis_of_rotation(2); 
         axis_of_rotation(3), 0, -axis_of_rotation(1); 
         -axis_of_rotation(2), axis_of_rotation(1), 0]; 
    R = eye(3) + sin(angle)*K + (1 - cos(angle))*(K^2);
    
    % Now, decompose the rotation matrix to extract the Euler angles
    Rx = -atan2(R(3,2), R(3,3)); % Rotation about X-axis
    %Ry = atan2(-R(3,1), sqrt(R(3,2)^2 + R(3,3)^2)); % Rotation about Y-axis
    denominator = max(sqrt(R(3,2)^2 + R(3,3)^2), eps); % Avoid division by zero
    Ry = -atan2(-R(3,1), denominator);

    
    
    Rz = 0; % No additional rotation needed around the Z-axis
end

== matlab function Main_C0_C3/TLF Flex/Latissimus Dorsi/WrappedMuscle4/MATLAB Function1 ==
  data: x1 input; length output; y1 input; z1 input; x2 input; y2 input; z2 input; Rx output; Ry output; Rz output
function [length, Rx, Ry, Rz] = computeCylinderParameters(x1, y1, z1, x2, y2, z2)
    % Compute the vector between the two frames
    vector = [x2 - x1, y2 - y1, z2 - z1];
    
    % Compute the length of the cylinder
    length = norm(vector);
    
    % Normalize the vector for direction
    unit_vector = vector / length;
    
    % Assume fixed axis (Z-axis)
    fixed_axis = [0, 0, 1];
    
    % Compute the axis of rotation (cross product)
    axis_of_rotation = cross(unit_vector, fixed_axis);
    
    % Avoid division by zero in case vectors are parallel
    if norm(axis_of_rotation) == 0
        % Handle case when the vectors are parallel
        if dot(unit_vector, fixed_axis) > 0
            % Vectors are aligned, no rotation needed
            Rx = 0;
            Ry = 0;
            Rz = 0;
        else
            % Vectors are in opposite directions, 180 degree rotation
            Rx = pi;
            Ry = 0;
            Rz = 0;
        end
        return;
    end
    
    % Normalize the axis of rotation
    axis_of_rotation = axis_of_rotation / norm(axis_of_rotation);
    
    % Compute the angle between vectors (dot product)
    cos_theta = dot(unit_vector, fixed_axis);
    
    % Clamp cos_theta to the range [-1, 1] to avoid domain errors in acos
    cos_theta = max(min(cos_theta, 1), -1);
    angle = acos(cos_theta);  % The angle between the vectors
    
    % Rodrigues' rotation formula to compute the rotation matrix
    K = [0, -axis_of_rotation(3), axis_of_rotation(2); 
         axis_of_rotation(3), 0, -axis_of_rotation(1); 
         -axis_of_rotation(2), axis_of_rotation(1), 0]; 
    R = eye(3) + sin(angle)*K + (1 - cos(angle))*(K^2);
    
    % Now, decompose the rotation matrix to extract the Euler angles
    Rx = -atan2(R(3,2), R(3,3)); % Rotation about X-axis
    %Ry = atan2(-R(3,1), sqrt(R(3,2)^2 + R(3,3)^2)); % Rotation about Y-axis
    denominator = max(sqrt(R(3,2)^2 + R(3,3)^2), eps); % Avoid division by zero
    Ry = -atan2(-R(3,1), denominator);

    
    
    Rz = 0; % No additional rotation needed around the Z-axis
end

== matlab function Main_C0_C3/TLF Flex/Latissimus Dorsi/WrappedMuscle1/MATLAB Function1 ==
  data: x1 input; length output; y1 input; z1 input; x2 input; y2 input; z2 input; Rx output; Ry output; Rz output
function [length, Rx, Ry, Rz] = computeCylinderParameters(x1, y1, z1, x2, y2, z2)
    % Compute the vector between the two frames
    vector = [x2 - x1, y2 - y1, z2 - z1];
    
    % Compute the length of the cylinder
    length = norm(vector);
    
    % Normalize the vector for direction
    unit_vector = vector / length;
    
    % Assume fixed axis (Z-axis)
    fixed_axis = [0, 0, 1];
    
    % Compute the axis of rotation (cross product)
    axis_of_rotation = cross(unit_vector, fixed_axis);
    
    % Avoid division by zero in case vectors are parallel
    if norm(axis_of_rotation) == 0
        % Handle case when the vectors are parallel
        if dot(unit_vector, fixed_axis) > 0
            % Vectors are aligned, no rotation needed
            Rx = 0;
            Ry = 0;
            Rz = 0;
        else
            % Vectors are in opposite directions, 180 degree rotation
            Rx = pi;
            Ry = 0;
            Rz = 0;
        end
        return;
    end
    
    % Normalize the axis of rotation
    axis_of_rotation = axis_of_rotation / norm(axis_of_rotation);
    
    % Compute the angle between vectors (dot product)
    cos_theta = dot(unit_vector, fixed_axis);
    
    % Clamp cos_theta to the range [-1, 1] to avoid domain errors in acos
    cos_theta = max(min(cos_theta, 1), -1);
    angle = acos(cos_theta);  % The angle between the vectors
    
    % Rodrigues' rotation formula to compute the rotation matrix
    K = [0, -axis_of_rotation(3), axis_of_rotation(2); 
         axis_of_rotation(3), 0, -axis_of_rotation(1); 
         -axis_of_rotation(2), axis_of_rotation(1), 0]; 
    R = eye(3) + sin(angle)*K + (1 - cos(angle))*(K^2);
    
    % Now, decompose the rotation matrix to extract the Euler angles
    Rx = -atan2(R(3,2), R(3,3)); % Rotation about X-axis
    %Ry = atan2(-R(3,1), sqrt(R(3,2)^2 + R(3,3)^2)); % Rotation about Y-axis
    denominator = max(sqrt(R(3,2)^2 + R(3,3)^2), eps); % Avoid division by zero
    Ry = -atan2(-R(3,1), denominator);

    
    
    Rz = 0; % No additional rotation needed around the Z-axis
end

== matlab function Main_C0_C3/TLF Flex/Latissimus Dorsi/WrappedMuscle1/MATLAB Function2 ==
  data: x1 input; length output; y1 input; z1 input; x2 input; y2 input; z2 input; Rx output; Ry output; Rz output
function [length, Rx, Ry, Rz] = computeCylinderParameters(x1, y1, z1, x2, y2, z2)
    % Compute the vector between the two frames
    vector = [x2 - x1, y2 - y1, z2 - z1];
    
    % Compute the length of the cylinder
    length = norm(vector);
    
    % Normalize the vector for direction
    unit_vector = vector / length;
    
    % Assume fixed axis (Z-axis)
    fixed_axis = [0, 0, 1];
    
    % Compute the axis of rotation (cross product)
    axis_of_rotation = cross(unit_vector, fixed_axis);
    
    % Avoid division by zero in case vectors are parallel
    if norm(axis_of_rotation) == 0
        % Handle case when the vectors are parallel
        if dot(unit_vector, fixed_axis) > 0
            % Vectors are aligned, no rotation needed
            Rx = 0;
            Ry = 0;
            Rz = 0;
        else
            % Vectors are in opposite directions, 180 degree rotation
            Rx = pi;
            Ry = 0;
            Rz = 0;
        end
        return;
    end
    
    % Normalize the axis of rotation
    axis_of_rotation = axis_of_rotation / norm(axis_of_rotation);
    
    % Compute the angle between vectors (dot product)
    cos_theta = dot(unit_vector, fixed_axis);
    
    % Clamp cos_theta to the range [-1, 1] to avoid domain errors in acos
    cos_theta = max(min(cos_theta, 1), -1);
    angle = acos(cos_theta);  % The angle between the vectors
    
    % Rodrigues' rotation formula to compute the rotation matrix
    K = [0, -axis_of_rotation(3), axis_of_rotation(2); 
         axis_of_rotation(3), 0, -axis_of_rotation(1); 
         -axis_of_rotation(2), axis_of_rotation(1), 0]; 
    R = eye(3) + sin(angle)*K + (1 - cos(angle))*(K^2);
    
    % Now, decompose the rotation matrix to extract the Euler angles
    Rx = -atan2(R(3,2), R(3,3)); % Rotation about X-axis
    %Ry = atan2(-R(3,1), sqrt(R(3,2)^2 + R(3,3)^2)); % Rotation about Y-axis
    denominator = max(sqrt(R(3,2)^2 + R(3,3)^2), eps); % Avoid division by zero
    Ry = -atan2(-R(3,1), denominator);

    
    
    Rz = 0; % No additional rotation needed around the Z-axis
end

== matlab function Main_C0_C3/TLF Flex/Latissimus Dorsi/WrappedMuscle2/MATLAB Function2 ==
  data: x1 input; length output; y1 input; z1 input; x2 input; y2 input; z2 input; Rx output; Ry output; Rz output
function [length, Rx, Ry, Rz] = computeCylinderParameters(x1, y1, z1, x2, y2, z2)
    % Compute the vector between the two frames
    vector = [x2 - x1, y2 - y1, z2 - z1];
    
    % Compute the length of the cylinder
    length = norm(vector);
    
    % Normalize the vector for direction
    unit_vector = vector / length;
    
    % Assume fixed axis (Z-axis)
    fixed_axis = [0, 0, 1];
    
    % Compute the axis of rotation (cross product)
    axis_of_rotation = cross(unit_vector, fixed_axis);
    
    % Avoid division by zero in case vectors are parallel
    if norm(axis_of_rotation) == 0
        % Handle case when the vectors are parallel
        if dot(unit_vector, fixed_axis) > 0
            % Vectors are aligned, no rotation needed
            Rx = 0;
            Ry = 0;
            Rz = 0;
        else
            % Vectors are in opposite directions, 180 degree rotation
            Rx = pi;
            Ry = 0;
            Rz = 0;
        end
        return;
    end
    
    % Normalize the axis of rotation
    axis_of_rotation = axis_of_rotation / norm(axis_of_rotation);
    
    % Compute the angle between vectors (dot product)
    cos_theta = dot(unit_vector, fixed_axis);
    
    % Clamp cos_theta to the range [-1, 1] to avoid domain errors in acos
    cos_theta = max(min(cos_theta, 1), -1);
    angle = acos(cos_theta);  % The angle between the vectors
    
    % Rodrigues' rotation formula to compute the rotation matrix
    K = [0, -axis_of_rotation(3), axis_of_rotation(2); 
         axis_of_rotation(3), 0, -axis_of_rotation(1); 
         -axis_of_rotation(2), axis_of_rotation(1), 0]; 
    R = eye(3) + sin(angle)*K + (1 - cos(angle))*(K^2);
    
    % Now, decompose the rotation matrix to extract the Euler angles
    Rx = -atan2(R(3,2), R(3,3)); % Rotation about X-axis
    %Ry = atan2(-R(3,1), sqrt(R(3,2)^2 + R(3,3)^2)); % Rotation about Y-axis
    denominator = max(sqrt(R(3,2)^2 + R(3,3)^2), eps); % Avoid division by zero
    Ry = -atan2(-R(3,1), denominator);

    
    
    Rz = 0; % No additional rotation needed around the Z-axis
end

== matlab function Main_C0_C3/TLF Flex/Latissimus Dorsi/WrappedMuscle3/MATLAB Function1 ==
  data: x1 input; length output; y1 input; z1 input; x2 input; y2 input; z2 input; Rx output; Ry output; Rz output
function [length, Rx, Ry, Rz] = computeCylinderParameters(x1, y1, z1, x2, y2, z2)
    % Compute the vector between the two frames
    vector = [x2 - x1, y2 - y1, z2 - z1];
    
    % Compute the length of the cylinder
    length = norm(vector);
    
    % Normalize the vector for direction
    unit_vector = vector / length;
    
    % Assume fixed axis (Z-axis)
    fixed_axis = [0, 0, 1];
    
    % Compute the axis of rotation (cross product)
    axis_of_rotation = cross(unit_vector, fixed_axis);
    
    % Avoid division by zero in case vectors are parallel
    if norm(axis_of_rotation) == 0
        % Handle case when the vectors are parallel
        if dot(unit_vector, fixed_axis) > 0
            % Vectors are aligned, no rotation needed
            Rx = 0;
            Ry = 0;
            Rz = 0;
        else
            % Vectors are in opposite directions, 180 degree rotation
            Rx = pi;
            Ry = 0;
            Rz = 0;
        end
        return;
    end
    
    % Normalize the axis of rotation
    axis_of_rotation = axis_of_rotation / norm(axis_of_rotation);
    
    % Compute the angle between vectors (dot product)
    cos_theta = dot(unit_vector, fixed_axis);
    
    % Clamp cos_theta to the range [-1, 1] to avoid domain errors in acos
    cos_theta = max(min(cos_theta, 1), -1);
    angle = acos(cos_theta);  % The angle between the vectors
    
    % Rodrigues' rotation formula to compute the rotation matrix
    K = [0, -axis_of_rotation(3), axis_of_rotation(2); 
         axis_of_rotation(3), 0, -axis_of_rotation(1); 
         -axis_of_rotation(2), axis_of_rotation(1), 0]; 
    R = eye(3) + sin(angle)*K + (1 - cos(angle))*(K^2);
    
    % Now, decompose the rotation matrix to extract the Euler angles
    Rx = -atan2(R(3,2), R(3,3)); % Rotation about X-axis
    %Ry = atan2(-R(3,1), sqrt(R(3,2)^2 + R(3,3)^2)); % Rotation about Y-axis
    denominator = max(sqrt(R(3,2)^2 + R(3,3)^2), eps); % Avoid division by zero
    Ry = -atan2(-R(3,1), denominator);

    
    
    Rz = 0; % No additional rotation needed around the Z-axis
end
